simulink model "PMSM_FOC_PowerGUI_Model"  (R2020b)
settings: Solver=FixedStepDiscrete  StartTime=0.0  StopTime=5  FixedStep=5e-7  RelTol=1e-3
model workspace (MAT data in the model file):
  wc = Simulink.Parameter
  wc.DataType = 'auto'
  wc.Dimensions = [0 0]
values from neighbouring files (symbols this model uses):
  Dead_Time = 0.0    [Hall_HSMO_FOC_Data.sldd]    (also in Hall_SMO_FOC_Data.sldd)
  Flux = 0.0109    [G474_FOC_HSMO.sldd]    (also in Hall_HSMO_FOC_Data.sldd = 0.00529276
  Ld = 0.000195185    [G474_FOC_HSMO.sldd]    (also in Hall_HSMO_FOC_Data.sldd = 0.0004
  Lq = 0.000195185    [G474_FOC_HSMO.sldd]    (also in Hall_HSMO_FOC_Data.sldd = 0.00045
  Pole_Pairs = 2.0    [Hall_HSMO_FOC_Data.sldd]    (also in Hall_SMO_FOC_Data.sldd)
  PWM_Frequency = 10000.0    [Hall_HSMO_FOC_Data.sldd]    (also in Hall_SMO_FOC_Data.sldd)
  R = 0.405    [Hall_HSMO_FOC_Data.sldd]    (also in Hall_SMO_FOC_Data.sldd = 0.4
undefined symbols (not defined in the file or in its folder): sigbuilder_block
libraries: powerlib x22, simulink x1
settings Model: DataDictionary=Hall_HSMO_FOC_Data.sldd  Creator=jt  LastModifiedBy=Administrator
settings DataIOCC: LimitDataPoints=on  SaveFormat=Array  ReturnWorkspaceOutputs=off
settings OptimizationCC: DefaultParameterBehavior=Inlined  UseDivisionForNetSlopeComputation=on  GainParamInheritBuiltInType=on  UseFloatMulNetSlope=on  InlineInvariantSignals=on  EnhancedBackFolding=on  PassReuseOutputArgsAs=Individual arguments  ZeroExternalMemoryAtStartup=off  ZeroInternalMemoryAtStartup=off  NoFixptDivByZeroProtection=on  EfficientFloat2IntCast=on  OptimizeBlockOrder=speed  DifferentSizesBufferReuse=on  OptimizationCustomize=off  EfficientTunableParamExpr=on
settings DebuggingCC: AlgebraicLoopMsg=none  MaxConsecutiveZCsMsg=none  SolverPrmCheckMsg=warning  ParameterTunabilityLossMsg=error  AllowSymbolicDim=off  SFUnexpectedBacktrackingDiag=warning  SFNoUnconditionalDefaultTransitionDiag=warning  SFExecutionAtInitializationDiag=none  ArithmeticOperatorsInVariantConditions=warning
settings HardwareCC: ProdBitPerPointer=32  ProdBitPerSizeT=32  ProdBitPerPtrDiffT=32  ProdLargestAtomicInteger=Long  ProdLargestAtomicFloat=Double  ProdEndianess=BigEndian  ProdWordSize=32  ProdLongLongMode=on  ProdHWDeviceType=Freescale->32-bit PowerPC
settings ModelReferenceCC: PropagateSignalLabelsOutOfModel=off
settings SFSimCC: SimUseLocalCustomCode=off  SimParseCustomCode=off  MATLABDynamicMemAlloc=off  CustomCodeUndefinedFunction=UseInterfaceOnly
settings RTWCC: Description=stm32 (Embedded Target)  SystemTargetFile=stm32.tlc  GenCodeOnly=on  TemplateMakefile=stm32.tmf  GenerateReport=on  RTWUseLocalCustomCode=off  IncludeHyperlinkInReport=on  GenerateTraceInfo=on  GenerateTraceReport=on  GenerateTraceReportSl=on  GenerateTraceReportSf=on  GenerateTraceReportEml=on  GenerateCodeMetricsReport=on
settings CodeAppCC: ForceParamTrailComments=on  IgnoreCustomStorageClasses=off  MaxIdLength=64  OperatorAnnotations=on  SimulinkDataObjDesc=on  SFDataObjDesc=on  CustomSymbolStrGlobalVar=rt$N$M  CustomSymbolStrType=$N$R$M  CustomSymbolStrFcn=$N$M$F  CustomSymbolStrMacro=$N$M  SimulinkBlockComments=off
settings STFCustomTargetCC: CodeReplacementLibrary=ARM CMSIS SIN COS  MultiwordLength=256  ParMdlRefBuildCompliant=on  ConcurrentExecutionCompliant=off  IncludeMdlTerminateFcn=off  CombineOutputUpdateFcns=on  ERTCustomFileBanners=on  SupportContinuousTime=off  SupportNonInlinedSFcns=off  RemoveResetFunc=on  MATLABClassNameForMDSCustomization=Simulink.SoftwareTarget.ERTCustomization  CPPClassGenCompliant=off  GRTInterface=off  SystemTargetFile=stm32.tlc
settings ERTTargetCC: CodeReplacementLibrary=ARM CMSIS SIN COS  CompOptLevelCompliant=off  ConcurrentExecutionCompliant=off  IncludeMdlTerminateFcn=off  ModelStepFunctionPrototypeControlCompliant=off  CPPClassGenCompliant=off  UseToolchainInfoCompliant=off  ExtModeStaticAllocSize=256  ExtModeMexFile=ext_serial_win32_comm  ExtModeMexArgs=0,1,115200,10  InlinedParameterPlacement=NonHierarchical  ERTSrcFileBannerTemplate=sourceFileTemplate.cgt  ERTHdrFileBannerTemplate=sourceFileTemplate.cgt  ERTDataSrcFileTemplate=sourceFileTemplate.cgt  ERTDataHdrFileTemplate=sourceFileTemplate.cgt  ERTCustomFileTemplate=customRoutineProcess.tlc
settings ConfigComp: CovMetricSettings=dw  CovSaveCumulativeToWorkspaceVar=on  CovSaveSingleToWorkspaceVar=on  CovExternalEMLEnable=off  CovSFcnEnable=off
settings SimscapeCC: SimscapeNormalizeSystem=off

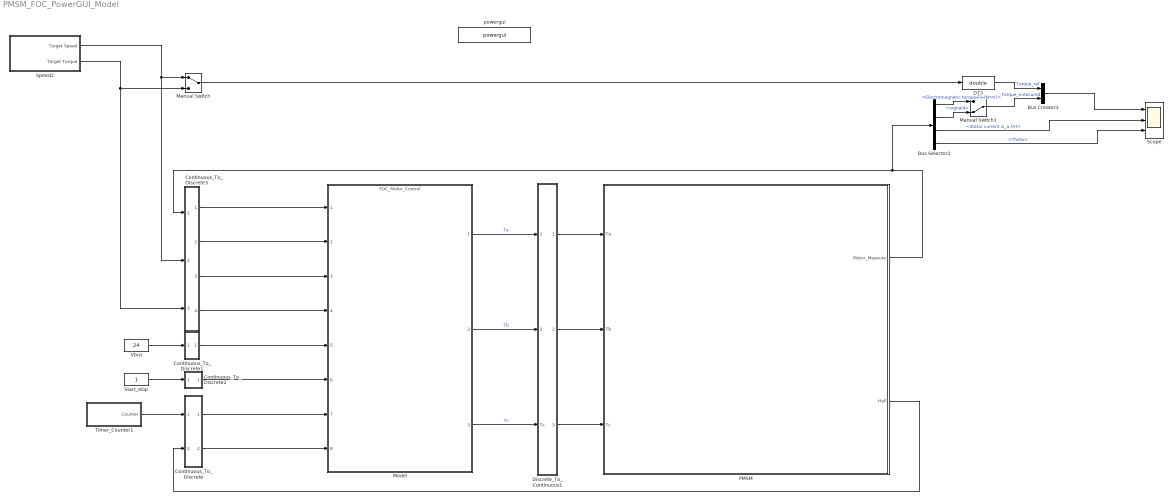
== system PMSM_FOC_PowerGUI_Model ==
  Bus Creator3 : BusCreator  Inputs=2
  Bus Selector2 : BusSelector  OutputSignals=Electromagnetic torque Te (N*m),signal4,Stator current is_a (A),Theta
  Continuous_To_Discrete : Subsystem
      mask Display: fprintf('C/D')
  Continuous_To_Discrete1 : Subsystem
      mask Display: fprintf('C/D')
  Continuous_To_Discrete2 : Subsystem
      mask Display: fprintf('C/D')
  Continuous_To_Discrete3 : Subsystem
      mask Display: fprintf('C/D')
  DT3 : DataTypeConversion  OutDataTypeStr=double
  Discrete_To_Continuous1 : Subsystem  Description=""
      mask Display: fprintf('D/C')
  Manual Switch : ManualSwitch
  Manual Switch1 : ManualSwitch  CurrentSetting=0
  Model : ModelReference  ModelNameDialog=FOC_Motor_Control.slx  SimulationMode=Normal  CodeInterface=Top model  ModelReferenceVersion=1.64
  PMSM : Subsystem
      mask Display: image('$imagefile'); % Use "Edit Image" on toolstrip to change.
  Scope : Scope  NumInputPorts=3
  Speed2 : Subsystem  Tag=STV Subsys  LoadFcn=sigbuilder_block('load');  StartFcn=sigbuilder_block('start');  StopFcn=sigbuilder_block('stop');  ClipboardFcn=sigbuilder_block('clipboard');  mask(Sigbuilder block){tuvar=[0:10]}
      mask help: Simulink:masks:SigbuilderBlock_MD
      mask init:
      | if ~strcmp(get_param(bdroot(gcbh),'SimulationStatus'),'stopped') tuvar = sigbuilder_block('maskInit'); end
      settings: CopyFcn=sigbuilder_block('copy');  DeleteFcn=sigbuilder_block('delete');  ModelCloseFcn=sigbuilder_block('modelClose');  PreSaveFcn=sigbuilder_block('preSave');  PauseFcn=sigbuilder_block('pause');  ContinueFcn=sigbuilder_block('continue');  NameChangeFcn=sigbuilder_block('namechange');  OpenFcn=sigbuilder_block('open',[48.5 0 906 449 ]);  CloseFcn=sigbuilder_block('close');
      mask Display: plot(0, 0, 100, 100,[2, 2, 32, 32, 2], [68, 8, 8, 68, 68],[32, 2], [38, 38], [32, 19, 2],[53, 60, 44], [32, 17, 17, 2],[16, 16, 31, 31]);txt = getActiveGroup(gcbh);text(2, 100, txt,'verticalAlignment', 'top');
  Start_stop : Constant  OutDataTypeStr=uint8
  Timer_Counter1 : Subsystem  TreatAsAtomicUnit=on
  Vbus : Constant  Value=24
  powergui : powerlib/powergui  Priority=1  SimulationMode=Discrete  SampleTime=5e-7  frequency=60  Iterations=50  frequencyindice=0  Pbase=100e6  ErrMax=1e-4  UnitsV=kV  UnitsW=MW  buscounter=0  FunctionMessages=off  echomessages=off  EnableUseOfTLC=off  CurrentSourceSwitches=off  DisableSnubberDevices=off  DisableRonSwitches=off  DisableVfSwitches=off  DisplayEquations=off  AutomaticDiscreteSolvers=off  SolverType=Tustin  Interpol=off  ExternalGateDelay=off  methode=off  Ts=0  x0status=blocks  SPID=off  SwTol=0  HookPort=off  NonlinearTolerance=1e-4  nMaxIteration=100  ContinueOnMaxIteration=off  RestoreLinks=warning  ResistiveCurrentMeasurement=off  Frange=[0:2:500]  Ylog=off  Xlog=on  ShowGrid=off  save=off  variable=ZData  structure=Iabc_FFT  ZoomFFT=off  StartTime=1  cycles=5  DisplayStyle=1  fundamental=13.333  FreqAxis=off  MaxFrequency=133.33  frequencyindicesteady=1  RmsSteady=1  display=off
  wires:
  Continuous_To_Discrete3/4(Theta) -> Model/4
  Manual Switch1/1 -> Bus Creator3/2  "Torque_measured"
  Model/1 -> Discrete_To_Continuous1/1(Ta)  "Ta"
  Continuous_To_Discrete3/2(Torque_ref) -> Model/2
  Bus Selector2/1 -> Manual Switch1/1  "<Electromagnetic torque Te (N*m)>"
  Bus Selector2/2 -> Manual Switch1/2  "<signal4>"
  Manual Switch/1 -> DT3/1
  Speed2/2(Target Torque) -> Continuous_To_Discrete3/3(Torque_command), Manual Switch/2
  DT3/1 -> Bus Creator3/1  "Torque_ref"
  Continuous_To_Discrete3/3(Phase_CurrentABC) -> Model/3
  Continuous_To_Discrete3/1(Speed_target) -> Model/1
  Model/2 -> Discrete_To_Continuous1/2(Tb)  "Tb"
  Bus Selector2/3 -> Scope/2  "<Stator current is_a (A)>"
  Discrete_To_Continuous1/3(T3) -> PMSM/3(Tc)
  Speed2/1(Target Speed) -> Continuous_To_Discrete3/2(Speed_Command), Manual Switch/1
  Bus Selector2/4 -> Scope/3  "<Theta>"
  Bus Creator3/1 -> Scope/1
  Model/3 -> Discrete_To_Continuous1/3(Tc)  "Tc"
  Discrete_To_Continuous1/2(T2) -> PMSM/2(Tb)
  Discrete_To_Continuous1/1(T1) -> PMSM/1(Ta)
  PMSM/1(Motor_Measure) -> Bus Selector2/1, Continuous_To_Discrete3/1(Motor_Measurements)
  Vbus/1 -> Continuous_To_Discrete1/1(Bus_Voltage)
  Continuous_To_Discrete1/1(Vbus) -> Model/5
  Continuous_To_Discrete2/1(Enable_Disable) -> Model/6
  Start_stop/1 -> Continuous_To_Discrete2/1(Start_stop)
  Timer_Counter1/1(Counter) -> Continuous_To_Discrete/1(Timer_counter)
  PMSM/2(Hall) -> Continuous_To_Discrete/2(Hall)
  Continuous_To_Discrete/1(Timer_Cnt) -> Model/7
  Continuous_To_Discrete/2(Hall_ABC) -> Model/8

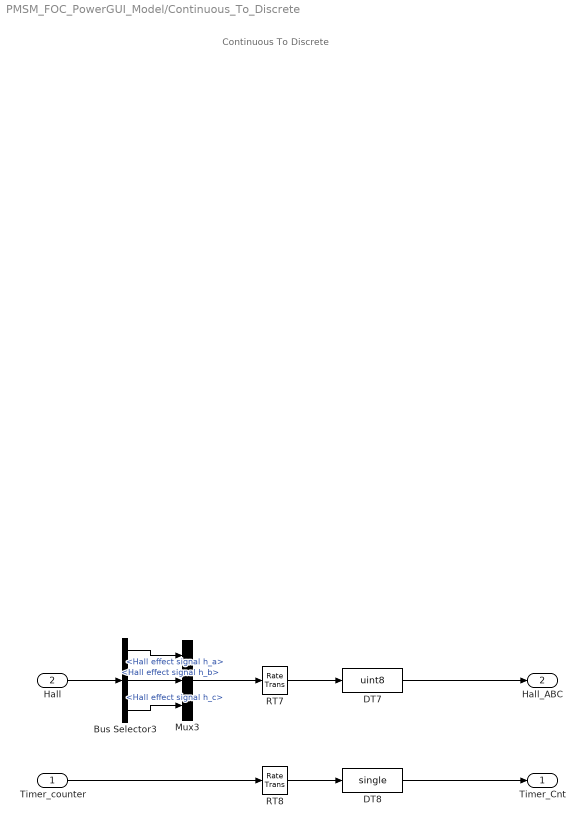
== system PMSM_FOC_PowerGUI_Model/Continuous_To_Discrete ==
  note: Continuous To Discrete
  Timer_counter : Inport
  Hall : Inport  Port=2
  Bus Selector3 : BusSelector  OutputSignals=Hall effect signal h_a,Hall effect signal h_b,Hall effect signal h_c
  DT7 : DataTypeConversion  OutDataTypeStr=uint8
  DT8 : DataTypeConversion  OutDataTypeStr=single
  Mux3 : Mux  Inputs=3
  RT7 : RateTransition  Integrity=off  OutPortSampleTime=1/PWM_Frequency
  RT8 : RateTransition  Integrity=off  OutPortSampleTime=1/PWM_Frequency
  Timer_Cnt : Outport  OutDataTypeStr=single
  Hall_ABC : Outport  Port=2
  wires:
  DT7/1 -> Hall_ABC/1
  Hall/1 -> Bus Selector3/1
  Mux3/1 -> RT7/1
  RT7/1 -> DT7/1
  Bus Selector3/1 -> Mux3/1  "<Hall effect signal h_a>"
  Bus Selector3/2 -> Mux3/2  "<Hall effect signal h_b>"
  RT8/1 -> DT8/1
  Timer_counter/1 -> RT8/1
  DT8/1 -> Timer_Cnt/1
  Bus Selector3/3 -> Mux3/3  "<Hall effect signal h_c>"

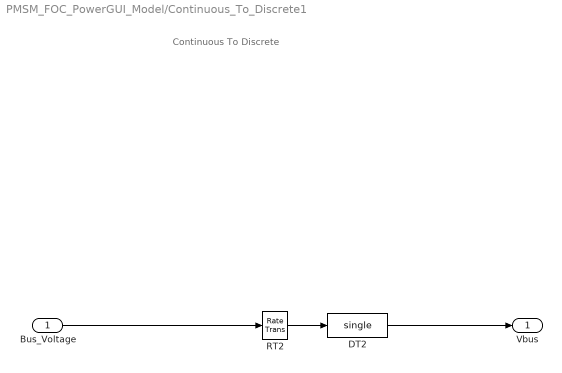
== system PMSM_FOC_PowerGUI_Model/Continuous_To_Discrete1 ==
  note: Continuous To Discrete
  Bus_Voltage : Inport
  DT2 : DataTypeConversion  OutDataTypeStr=single
  RT2 : RateTransition  Integrity=off
  Vbus : Outport
  wires:
  Bus_Voltage/1 -> RT2/1
  RT2/1 -> DT2/1
  DT2/1 -> Vbus/1

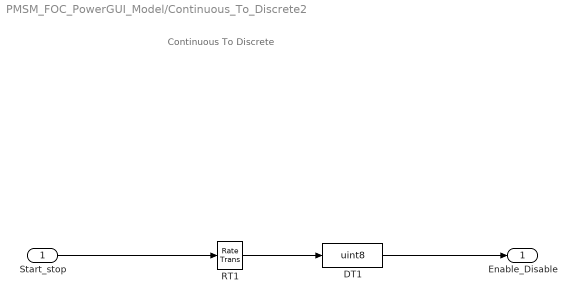
== system PMSM_FOC_PowerGUI_Model/Continuous_To_Discrete2 ==
  note: Continuous To Discrete
  Start_stop : Inport
  DT1 : DataTypeConversion  OutDataTypeStr=uint8
  RT1 : RateTransition  Integrity=off
  Enable_Disable : Outport
  wires:
  DT1/1 -> Enable_Disable/1
  RT1/1 -> DT1/1
  Start_stop/1 -> RT1/1

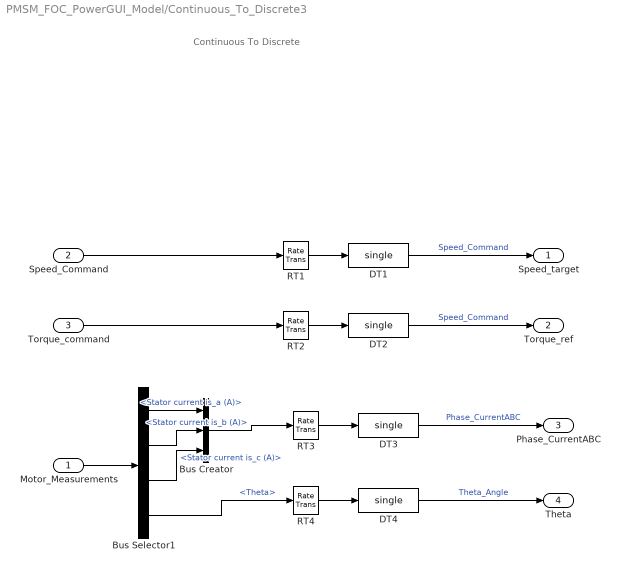
== system PMSM_FOC_PowerGUI_Model/Continuous_To_Discrete3 ==
  note: Continuous To Discrete
  Motor_Measurements : Inport
  Speed_Command : Inport  Port=2
  Torque_command : Inport  Port=3
  Bus Creator : BusCreator  Inputs=3
  Bus Selector1 : BusSelector  OutputSignals=Stator current is_a (A),Stator current is_b (A),Stator current is_c (A),Theta
  DT{1..4} (4 alike) : DataTypeConversion  OutDataTypeStr=single
  RT{1..4} (4 alike) : RateTransition  Integrity=off
  Speed_target : Outport
  Torque_ref : Outport  Port=2
  Phase_CurrentABC : Outport  Port=3  PortDimensions=3
  Theta : Outport  Port=4
  wires:
  DT1/1 -> Speed_target/1  "Speed_Command"
  RT1/1 -> DT1/1
  RT3/1 -> DT3/1
  Motor_Measurements/1 -> Bus Selector1/1
  Speed_Command/1 -> RT1/1
  RT4/1 -> DT4/1
  DT4/1 -> Theta/1  "Theta_Angle"
  DT3/1 -> Phase_CurrentABC/1  "Phase_CurrentABC"
  Bus Selector1/4 -> RT4/1  "<Theta>"
  Torque_command/1 -> RT2/1
  RT2/1 -> DT2/1
  DT2/1 -> Torque_ref/1  "Speed_Command"
  Bus Creator/1 -> RT3/1
  Bus Selector1/1 -> Bus Creator/1  "<Stator current is_a (A)>"
  Bus Selector1/2 -> Bus Creator/2  "<Stator current is_b (A)>"
  Bus Selector1/3 -> Bus Creator/3  "<Stator current is_c (A)>"

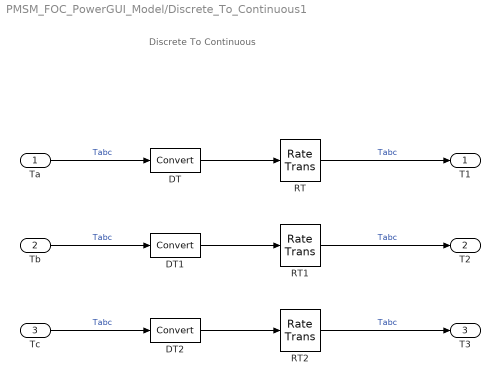
== system PMSM_FOC_PowerGUI_Model/Discrete_To_Continuous1 ==
  note: Discrete To Continuous
  Ta : Inport
  Tb : Inport  Port=2
  Tc : Inport  Port=3
  DT : DataTypeConversion
  DT1 : DataTypeConversion
  DT2 : DataTypeConversion
  RT : RateTransition  Integrity=off
  RT1 : RateTransition  Integrity=off
  RT2 : RateTransition  Integrity=off
  T1 : Outport
  T2 : Outport  Port=2
  T3 : Outport  Port=3
  wires:
  DT/1 -> RT/1
  Ta/1 -> DT/1  "Tabc"
  DT1/1 -> RT1/1
  Tb/1 -> DT1/1  "Tabc"
  DT2/1 -> RT2/1
  Tc/1 -> DT2/1  "Tabc"
  RT/1 -> T1/1  "Tabc"
  RT1/1 -> T2/1  "Tabc"
  RT2/1 -> T3/1  "Tabc"

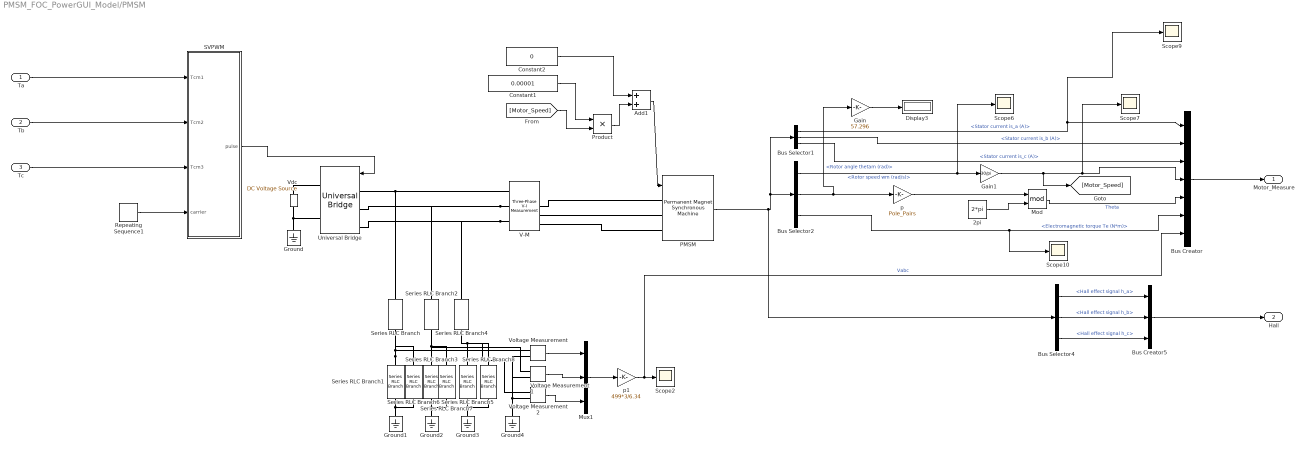
== system PMSM_FOC_PowerGUI_Model/PMSM ==
  Ta : Inport
  Tb : Inport  Port=2
  Tc : Inport  Port=3
  2pi : Constant  Value=2*pi
  Add1 : Sum
  Bus Creator : BusCreator  Inputs=7
  Bus Creator5 : BusCreator  Inputs=3
  Bus Selector1 : BusSelector  OutputSignals=Stator current is_a (A),Stator current is_b (A),Stator current is_c (A)
  Bus Selector2 : BusSelector  OutputSignals=Rotor speed wm (rad/s),Rotor angle thetam (rad),Electromagnetic torque Te (N*m)
  Bus Selector4 : BusSelector  OutputSignals=Hall effect signal h_a,Hall effect signal h_b,Hall effect signal h_c
  Constant1 : Constant  Value=0.00001
  Constant2 : Constant  Value=0
  Display3 : Display
  Gain : Gain  Gain=57.296
  Gain1 : Gain  Gain=30/pi  OutDataTypeStr=Inherit: Same as input  ParamDataTypeStr=Inherit: Same as input
  Ground{,1..4} (5 alike) : powerlib/Elements/Ground  LConnTagsString=a
  Mod : Math  Operator=mod  SaturateOnIntegerOverflow=on
  Mux1 : Mux  Inputs=3
  PMSM : powerlib/Machines/Permanent Magnet Synchronous Machine  NbPhases=3  FluxDistribution=Sinusoidal  RotorType=Salient-pole  MechanicalLoad=Torque Tm  PresetModel=No  ShowDetailedParameters=on  MeasurementBus=off  Resistance=R  Inductance=8.5e-3  dqInductances=[Ld Lq]  La=0.015  MachineConstant=Flux linkage established by magnets (V.s)  Flux=Flux  VoltageCst=9.4612  TorqueCst=0.078244  Flat=120  Mechanical=[1e-4 0 Pole_Pairs 0]  PolePairs=3  InitialConditions=[0,0,0,0]  InitialConditions5ph=[0 0 0 0 0 0]  RefAngle=Aligned with phase A axis (original Park)  IterativeDiscreteModel=Trapezoidal non iterative  TsBlock=-1  TsPowergui=0
  Product : Product
  Repeating Sequence1 : simulink/Sources/Repeating Sequence  rep_seq_t=[0 (1/PWM_Frequency/2) 1/PWM_Frequency]  rep_seq_y=[0 0.00005*83990000 0]
  SVPWM : Subsystem  TreatAsAtomicUnit=on
  Scope{2,6..7,9..10} (5 alike) : Scope
  Series RLC Branch : powerlib/Elements/Series RLC Branch  LConnTagsString=__new0  RConnTagsString=__new0  BranchType=R  Resistance=499*1000*3  Inductance=1e-3  SetiL0=off  InitialCurrent=0  Capacitance=1e-6  Setx0=off  InitialVoltage=0  Measurements=None
  Series RLC Branch1 : powerlib/Elements/Series RLC Branch  LConnTagsString=__new0  RConnTagsString=__new0  BranchType=R  Resistance=6.34*1000  Inductance=1e-3  SetiL0=off  InitialCurrent=0  Capacitance=1e-6  Setx0=off  InitialVoltage=0  Measurements=None
  Series RLC Branch2 : powerlib/Elements/Series RLC Branch  LConnTagsString=__new0  RConnTagsString=__new0  BranchType=R  Resistance=499*3*1000  Inductance=1e-3  SetiL0=off  InitialCurrent=0  Capacitance=1e-6  Setx0=off  InitialVoltage=0  Measurements=None
  Series RLC Branch3 : powerlib/Elements/Series RLC Branch  LConnTagsString=__new0  RConnTagsString=__new0  BranchType=R  Resistance=6.34*1000  Inductance=1e-3  SetiL0=off  InitialCurrent=0  Capacitance=1e-6  Setx0=off  InitialVoltage=0  Measurements=None
  Series RLC Branch4 : powerlib/Elements/Series RLC Branch  LConnTagsString=__new0  RConnTagsString=__new0  BranchType=R  Resistance=499*3*1000  Inductance=1e-3  SetiL0=off  InitialCurrent=0  Capacitance=1e-6  Setx0=off  InitialVoltage=0  Measurements=None
  Series RLC Branch5 : powerlib/Elements/Series RLC Branch  LConnTagsString=__new0  RConnTagsString=__new0  BranchType=R  Resistance=6.34*1000  Inductance=1e-3  SetiL0=off  InitialCurrent=0  Capacitance=1e-6  Setx0=off  InitialVoltage=0  Measurements=None
  Series RLC Branch6 : powerlib/Elements/Series RLC Branch  LConnTagsString=__new0  RConnTagsString=__new0  BranchType=C  Resistance=6.34  Inductance=1e-3  SetiL0=off  InitialCurrent=0  Capacitance=0.047/1000000  Setx0=off  InitialVoltage=0  Measurements=None
  Series RLC Branch7 : powerlib/Elements/Series RLC Branch  LConnTagsString=__new0  RConnTagsString=__new0  BranchType=C  Resistance=6.34  Inductance=1e-3  SetiL0=off  InitialCurrent=0  Capacitance=0.047/1000000  Setx0=off  InitialVoltage=0  Measurements=None
  Series RLC Branch8 : powerlib/Elements/Series RLC Branch  LConnTagsString=__new0  RConnTagsString=__new0  BranchType=C  Resistance=6.34  Inductance=1e-3  SetiL0=off  InitialCurrent=0  Capacitance=0.047/1000000  Setx0=off  InitialVoltage=0  Measurements=None
  Universal Bridge : powerlib/Power Electronics/Universal Bridge  Arms=3  SnubberResistance=1e5  SnubberCapacitance=inf  Device=IGBT / Diodes  Ron=1e-3  Lon=0  ForwardVoltages="[  0  0  ]"  ForwardVoltage=0  GTOparameters=[ 10e-6 , 20e-6 ]  IGBTparameters=[ 1e-6 , 2e-6 ]  Measurements=None  Measurements_2=None  converterType=Rectifier
  V-M : powerlib/Measurements/Three-Phase V-I Measurement  VoltageMeasurement=phase-to-ground  SetLabelV=off  LabelV=Vabc  Vpu=off  VpuLL=off  CurrentMeasurement=yes  SetLabelI=off  LabelI=Iabc  Ipu=off  Pbase=100e6  Vbase=500e3  OutputType=Complex  PhasorSimulation=off  PSBequivalent=0
  "Vdc " : powerlib/Electrical Sources/DC Voltage Source  Amplitude=350  Measurements=None
  Voltage Measurement : powerlib/Measurements/Voltage Measurement  PhasorSimulation=off  OutputType=Complex  PSBequivalent=0
  Voltage Measurement1 : powerlib/Measurements/Voltage Measurement  PhasorSimulation=off  OutputType=Complex  PSBequivalent=0
  Voltage Measurement2 : powerlib/Measurements/Voltage Measurement  PhasorSimulation=off  OutputType=Complex  PSBequivalent=0
  p : Gain  Gain=Pole_Pairs  OutDataTypeStr=Inherit: Same as input  ParamDataTypeStr=Inherit: Same as input
  p1 : Gain  Gain=499*3/6.34  OutDataTypeStr=Inherit: Same as input  ParamDataTypeStr=Inherit: Same as input
  Motor_Measure : Outport
  Hall : Outport  Port=2
  wires:
  Repeating Sequence1/1 -> SVPWM/4(carrier)
  Mod/1 -> Bus Creator/5  "Theta"
  p1/1 -> Bus Creator/7, Scope2/1  "Vabc"
  Voltage Measurement2/1 -> Mux1/3
  Voltage Measurement/1 -> Mux1/1
  Mux1/1 -> p1/1
  2pi/1 -> Mod/2
  Voltage Measurement1/1 -> Mux1/2
  p/1 -> Mod/1
  Bus Selector2/2 -> Gain/1, p/1  "<Rotor angle thetam (rad)>"
  Bus Selector1/1 -> Scope9/1, Bus Creator/1  "<Stator current is_a (A)>"
  Bus Selector2/3 -> Scope10/1, Bus Creator/6  "<Electromagnetic torque Te (N*m)>"
  Bus Selector1/2 -> Bus Creator/2  "<Stator current is_b (A)>"
  Bus Selector2/1 -> Scope6/1, Gain1/1  "<Rotor speed wm (rad/s)>"
  Gain1/1 -> [Motor_Speed], Scope7/1, Bus Creator/4
  Bus Creator/1 -> Motor_Measure/1
  Bus Selector1/3 -> Bus Creator/3  "<Stator current is_c (A)>"
  Gain/1 -> Display3/1
  Ta/1 -> SVPWM/1(Tcm1)
  Tb/1 -> SVPWM/2(Tcm2)
  Tc/1 -> SVPWM/3(Tcm3)
  SVPWM/1(pulse) -> Universal Bridge/1
  [Motor_Speed] -> Product/2
  Constant1/1 -> Product/1
  Product/1 -> Add1/2
  Add1/1 -> PMSM/1
  Bus Selector4/2 -> Bus Creator5/2  "<Hall effect signal h_b>"
  Bus Selector4/1 -> Bus Creator5/1  "<Hall effect signal h_a>"
  Bus Selector4/3 -> Bus Creator5/3  "<Hall effect signal h_c>"
  PMSM/1 -> Bus Selector4/1, Bus Selector2/1, Bus Selector1/1
  Bus Creator5/1 -> Hall/1
  Constant2/1 -> Add1/1
  connections:
  "Vdc "/RConn1 -- Universal Bridge/RConn1
  Universal Bridge/RConn2 -- "Vdc "/LConn1 -- Ground/LConn1
  Series RLC Branch/RConn1 -- Universal Bridge/LConn1 -- V-M/LConn1
  V-M/LConn2 -- Universal Bridge/LConn2 -- Series RLC Branch2/RConn1
  V-M/LConn3 -- Universal Bridge/LConn3 -- Series RLC Branch4/RConn1
  Series RLC Branch8/RConn1 -- Series RLC Branch5/RConn1 -- Ground3/LConn1
  Ground4/LConn1 -- Voltage Measurement2/LConn2 -- Voltage Measurement/LConn2 -- Voltage Measurement1/LConn2
  Series RLC Branch2/LConn1 -- Series RLC Branch7/LConn1 -- Voltage Measurement1/LConn1 -- Series RLC Branch3/LConn1
  Series RLC Branch4/LConn1 -- Voltage Measurement2/LConn1 -- Series RLC Branch8/LConn1 -- Series RLC Branch5/LConn1
  Series RLC Branch6/RConn1 -- Series RLC Branch1/RConn1 -- Ground1/LConn1
  Series RLC Branch1/LConn1 -- Voltage Measurement/LConn1 -- Series RLC Branch/LConn1 -- Series RLC Branch6/LConn1
  Series RLC Branch7/RConn1 -- Series RLC Branch3/RConn1 -- Ground2/LConn1
  V-M/RConn1 -- PMSM/LConn1
  V-M/RConn2 -- PMSM/LConn2
  V-M/RConn3 -- PMSM/LConn3

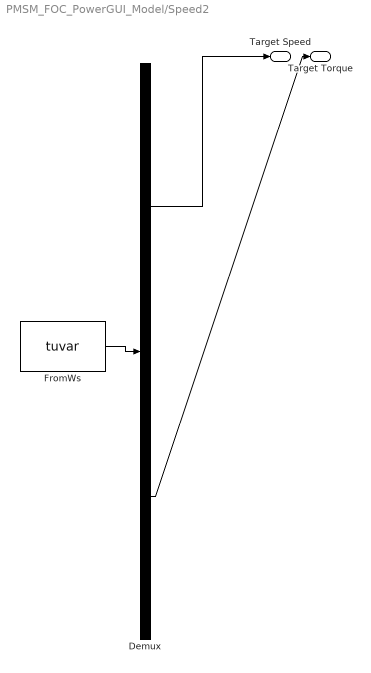
== system PMSM_FOC_PowerGUI_Model/Speed2 ==
  Demux : Demux  Tag=STV Demux  Outputs=2
      settings: DisplayOption=none
  FromWs : FromWorkspace  Tag=STV FromWs  VariableName=tuvar
      SigBuilderData=|
      | common.afterFinalStr = 'Extrapolate'
      | common.sampleTime = 0
      | dataSet.timeRange = [0 10]
      | dataSet.name = 'Target Speed'
      | sbobj.Groups.Name = 'Target Speed'
      | sbobj.Groups.Signals(1).Name = 'Target Speed'
      | sbobj.Groups.Signals(1).XData = [0 0.35 0.35 0.78 0.78 1.14 1.14 10]
      | sbobj.Groups.Signals(1).YData = [1500 1500 2000 2000 3020 3020 1995 1995]
      | sbobj.Groups.Signals(2).Name = 'Target Torque'
      | sbobj.Groups.Signals(2).XData = [0 4 4 6 6 10]
      | sbobj.Groups.Signals(2).YData = [0 0 1 1 0 0]
  Target Speed : Outport  Tag=STV Outport
  Target Torque : Outport  Tag=STV Outport  Port=2
  wires:
  FromWs/1 -> Demux/1
  Demux/1 -> Target Speed/1
  Demux/2 -> Target Torque/1

== system PMSM_FOC_PowerGUI_Model/Timer_Counter1 ==
  Add2 : Sum
  Constant3 : Constant  OutDataTypeStr=single
  Memory : Memory  InheritSampleTime=on
  Counter : Outport
  wires:
  Add2/1 -> Counter/1, Memory/1
  Constant3/1 -> Add2/1
  Memory/1 -> Add2/2

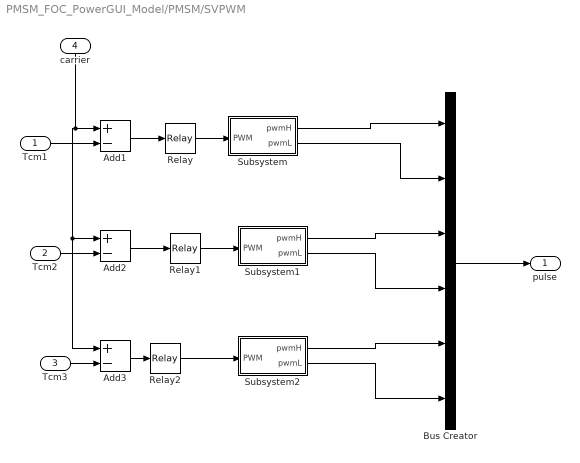
== system PMSM_FOC_PowerGUI_Model/PMSM/SVPWM ==
  Tcm1 : Inport
  Tcm2 : Inport  Port=2
  Tcm3 : Inport  Port=3
  carrier : Inport  Port=4
  Add1 : Sum  Inputs=+-
  Add2 : Sum  Inputs=+-
  Add3 : Sum  Inputs=+-
  Bus Creator : BusCreator  Inputs=6
  Relay : Relay
  Relay1 : Relay
  Relay2 : Relay
  Subsystem : Subsystem
  Subsystem1 : Subsystem
  Subsystem2 : Subsystem
  pulse : Outport
  wires:
  carrier/1 -> Add1/1, Add2/1, Add3/1
  Tcm2/1 -> Add2/2
  Tcm3/1 -> Add3/2
  Add3/1 -> Relay2/1
  Add2/1 -> Relay1/1
  Add1/1 -> Relay/1
  Tcm1/1 -> Add1/2
  Relay2/1 -> Subsystem2/1(PWM)
  Relay/1 -> Subsystem/1(PWM)
  Relay1/1 -> Subsystem1/1(PWM)
  Bus Creator/1 -> pulse/1
  Subsystem/1(pwmH) -> Bus Creator/1
  Subsystem/2(pwmL) -> Bus Creator/2
  Subsystem1/1(pwmH) -> Bus Creator/3
  Subsystem1/2(pwmL) -> Bus Creator/4
  Subsystem2/1(pwmH) -> Bus Creator/5
  Subsystem2/2(pwmL) -> Bus Creator/6

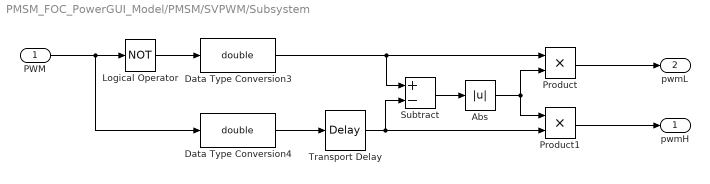
== system PMSM_FOC_PowerGUI_Model/PMSM/SVPWM/Subsystem ==
  PWM : Inport
  Abs : Abs
  Data Type Conversion3 : DataTypeConversion  OutDataTypeStr=double
  Data Type Conversion4 : DataTypeConversion  OutDataTypeStr=double
  Logical Operator : Logic  Operator=NOT  AllPortsSameDT=off  OutDataTypeStr=boolean
  Product : Product
  Product1 : Product
  Subtract : Sum  Inputs=+-
  Transport Delay : TransportDelay  DelayTime=Dead_Time
  pwmH : Outport
  pwmL : Outport  Port=2
  wires:
  PWM/1 -> Data Type Conversion4/1, Logical Operator/1
  Subtract/1 -> Abs/1
  Transport Delay/1 -> Subtract/2, Product1/2
  Abs/1 -> Product1/1, Product/2
  Data Type Conversion3/1 -> Subtract/1, Product/1
  Product1/1 -> pwmH/1
  Product/1 -> pwmL/1
  Logical Operator/1 -> Data Type Conversion3/1
  Data Type Conversion4/1 -> Transport Delay/1

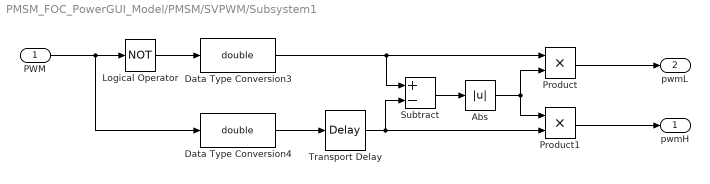
== system PMSM_FOC_PowerGUI_Model/PMSM/SVPWM/Subsystem1 ==
  PWM : Inport
  Abs : Abs
  Data Type Conversion3 : DataTypeConversion  OutDataTypeStr=double
  Data Type Conversion4 : DataTypeConversion  OutDataTypeStr=double
  Logical Operator : Logic  Operator=NOT  AllPortsSameDT=off  OutDataTypeStr=boolean
  Product : Product
  Product1 : Product
  Subtract : Sum  Inputs=+-
  Transport Delay : TransportDelay  DelayTime=Dead_Time
  pwmH : Outport
  pwmL : Outport  Port=2
  wires:
  PWM/1 -> Data Type Conversion4/1, Logical Operator/1
  Subtract/1 -> Abs/1
  Transport Delay/1 -> Subtract/2, Product1/2
  Abs/1 -> Product1/1, Product/2
  Data Type Conversion3/1 -> Subtract/1, Product/1
  Product1/1 -> pwmH/1
  Product/1 -> pwmL/1
  Logical Operator/1 -> Data Type Conversion3/1
  Data Type Conversion4/1 -> Transport Delay/1

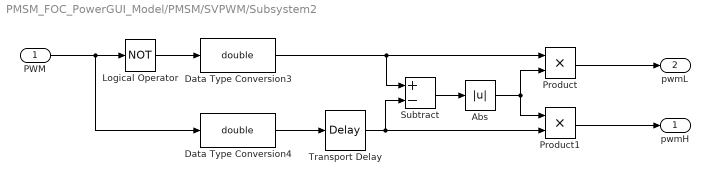
== system PMSM_FOC_PowerGUI_Model/PMSM/SVPWM/Subsystem2 ==
  PWM : Inport
  Abs : Abs
  Data Type Conversion3 : DataTypeConversion  OutDataTypeStr=double
  Data Type Conversion4 : DataTypeConversion  OutDataTypeStr=double
  Logical Operator : Logic  Operator=NOT  AllPortsSameDT=off  OutDataTypeStr=boolean
  Product : Product
  Product1 : Product
  Subtract : Sum  Inputs=+-
  Transport Delay : TransportDelay  DelayTime=Dead_Time
  pwmH : Outport
  pwmL : Outport  Port=2
  wires:
  PWM/1 -> Data Type Conversion4/1, Logical Operator/1
  Subtract/1 -> Abs/1
  Transport Delay/1 -> Subtract/2, Product1/2
  Abs/1 -> Product1/1, Product/2
  Data Type Conversion3/1 -> Subtract/1, Product/1
  Product1/1 -> pwmH/1
  Product/1 -> pwmL/1
  Logical Operator/1 -> Data Type Conversion3/1
  Data Type Conversion4/1 -> Transport Delay/1
